simulink library "csu_lpc_landing_pre_coast_lib"  (R2015b)
settings: Solver=ode45  StartTime=0.0  StopTime=10.0  RelTol=1e-3
undefined symbols (not defined in the file or in its folder): DiscIntNeverNeededParam, lpc_pre_coast_time
libraries: util_info_lib x1
settings Model: Creator=escrane  LastModifiedBy=jimkaidy
settings DataIOCC: SaveFormat=Array
settings DebuggingCC: UnderspecifiedInitializationDetection=Classic  MergeDetectMultiDrivingBlocksExec=none  SolverPrmCheckMsg=warning
settings HardwareCC: ProdBitPerPointer=32  ProdLargestAtomicFloat=None  ProdIntDivRoundTo=Undefined  ProdEndianess=Unspecified  ProdWordSize=32  ProdHWDeviceType=32-bit Generic
settings GRTTargetCC: GeneratePreprocessorConditionals=Disable all
settings ConfigComp: CovModelRefEnable=Off  CovSFcnEnable=off

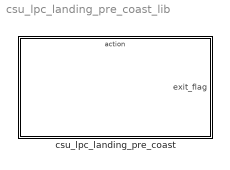
== system csu_lpc_landing_pre_coast_lib ==
  csu_lpc_landing_pre_coast : Subsystem  TreatAsAtomicUnit=on

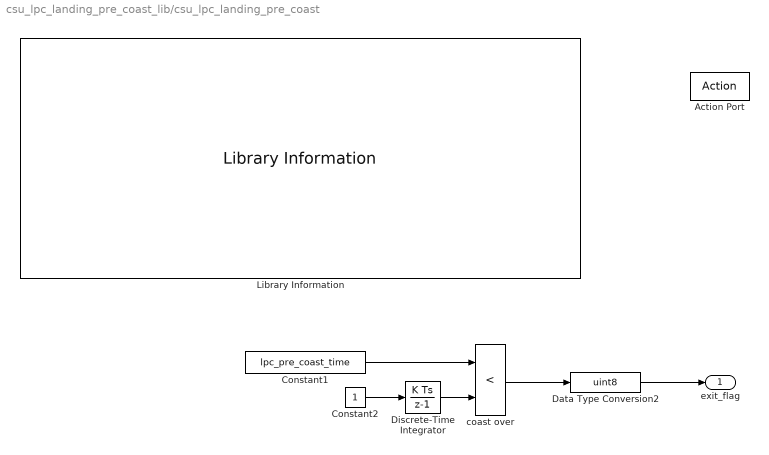
== system csu_lpc_landing_pre_coast_lib/csu_lpc_landing_pre_coast ==
  Action Port : ActionPort
  Constant1 : Constant  Value=lpc_pre_coast_time
  Constant2 : Constant
  Data Type Conversion2 : DataTypeConversion  OutDataTypeStr=uint8
  Discrete-Time Integrator : DiscreteIntegrator  SampleTime=-1  ICPrevOutput=DiscIntNeverNeededParam  ICPrevScaledInput=DiscIntNeverNeededParam
  Library Information : util_info_lib/Library Information  owner='NONE'
  coast over : RelationalOperator  Operator=<  OutDataTypeStr=boolean
  exit_flag : Outport  InitialOutput=0
  wires:
  Data Type Conversion2/1 -> exit_flag/1
  Constant1/1 -> coast over/1
  Discrete-Time Integrator/1 -> coast over/2
  Constant2/1 -> Discrete-Time Integrator/1
  coast over/1 -> Data Type Conversion2/1
